simulink model "sampleModel191"  (R2021b)
settings: Solver=VariableStepAuto  StartTime=0.0  StopTime=10.0  RelTol=1e-3
libraries: simulink x2
settings Model: Creator=user  LastModifiedBy=user

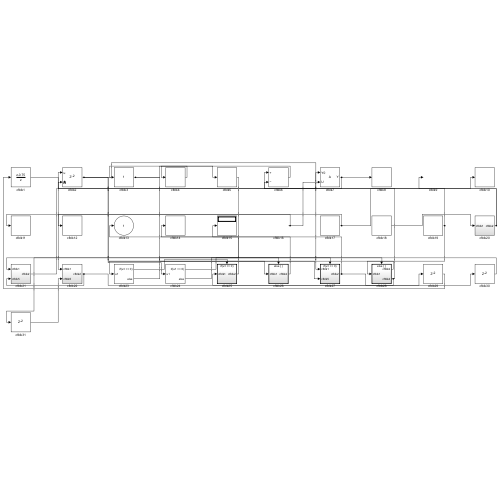
[thumbnail: Simulink's stored preview of the top-level diagram]
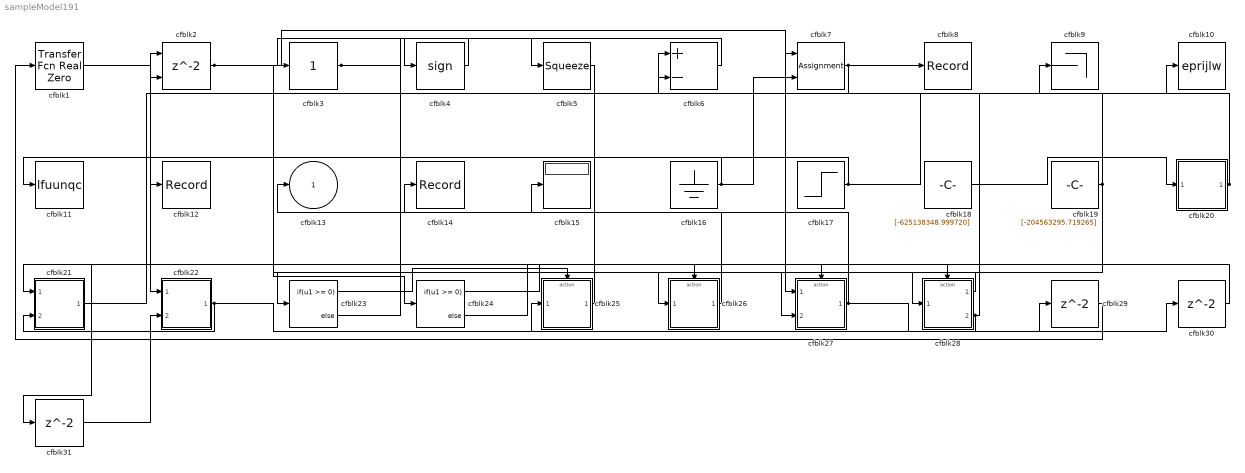
== system sampleModel191 ==
  cfblk1 : simulink/Discrete/Transfer Fcn Real Zero  ZeroZ=0.75  ICPrevInput=0.0  DoSatur=off
      settings: SourceProductBaseCode=SL
  cfblk10 : ToWorkspace  VariableName=eprijlw  SaveFormat=Timeseries  SampleTime=-1
  cfblk11 : ToWorkspace  VariableName=lfuunqc  SaveFormat=Timeseries  SampleTime=-1
  cfblk12 : Record  FileSettingsInternal="{\"entries\":[{\"content\":{\"excelSettings\":{\"content\":{},\"type\":\"Streamout.ExcelSettings\"}},\"type\":\"Streamout.FileSettingStorage\",\"uuid\":\"be9789c7-0946-41dc-ba80-fdfecf057616\"}],\"packageUris\":[\"http://schema.mathworks.com/mf0/streamout_blocks/R2020a\"],\"version\":\"1.0\"}"  SignalsInternal="{\"entries\":[{\"content\":{\"signals\":[{\"content\":{\"blockPath\":[\"sampleModel191/cfblk12\"],\"channel\":[],\"dimensions\":[1],\"domain\":\"sampleModel191/cfblk12\",\"lineColor\":\"#77ac30\",\"plots\":[1],\"port\":1,\"sid\":[\"\"],\"signalID\":7140,\"signalName\":\"cfblk17\"},\"type\":\"RecordBlkView.Signal\",\"uuid\":\"3feb5f82-e466-445f-8270-1e8679e3d33b\"}]},\"type\":\"RecordBlkView.InputSignals\",\"uuid\":\"5d828b83-df96-49b2-94c2-6ae34a61bf7d\"}],\"packageUris\":[\"http://schema.mathworks.com/mf0/streamout_blocks/R2020a\"],\"version\":\"1.0\"}"  VisualizationBindings="{\"sparklinesplugin\":{\"info\":[{\"bindingParametersList\":[],\"subplotID\":1}]}}"
  cfblk14 : Record  FileSettingsInternal="{\"entries\":[{\"content\":{\"excelSettings\":{\"content\":{},\"type\":\"Streamout.ExcelSettings\"}},\"type\":\"Streamout.FileSettingStorage\",\"uuid\":\"e2498147-d1e1-4463-9837-c808039952d8\"}],\"packageUris\":[\"http://schema.mathworks.com/mf0/streamout_blocks/R2020a\"],\"version\":\"1.0\"}"  SignalsInternal="{\"entries\":[{\"content\":{\"signals\":[{\"content\":{\"blockPath\":[\"sampleModel191/cfblk14\"],\"channel\":[],\"dimensions\":[1],\"domain\":\"sampleModel191/cfblk14\",\"lineColor\":\"#edb120\",\"plots\":[1],\"port\":1,\"sid\":[\"\"],\"signalID\":7132,\"signalName\":\"cfblk25\"},\"type\":\"RecordBlkView.Signal\",\"uuid\":\"96d69e8b-c9dd-4632-86a4-9ef49d9a27d5\"}]},\"type\":\"RecordBlkView.InputSignals\",\"uuid\":\"17047321-6578-4322-be57-9c84a47ba275\"}],\"packageUris\":[\"http://schema.mathworks.com/mf0/streamout_blocks/R2020a\"],\"version\":\"1.0\"}"  VisualizationBindings="{\"sparklinesplugin\":{\"info\":[{\"bindingParametersList\":[],\"subplotID\":1}]}}"
  cfblk15 : Display
  cfblk16 : Ground
  cfblk17 : Step  Time=[11.000000]  Before=[445527667.725951]  After=[-252859869.067699]  SampleTime=0
  cfblk18 : Constant  Value=[-625138348.999720]  SampleTime=1
  cfblk19 : Constant  Value=[-204563295.719265]  SampleTime=1
  cfblk2 : Delay  ShowEnablePort=on  SampleTime=1
      settings: InputPortMap=u0,e6
  cfblk20 : Subsystem
  cfblk21 : Subsystem
  cfblk22 : Subsystem
  cfblk23 : If  IfExpression=u1 >= 0  SampleTime=1
  cfblk24 : If  IfExpression=u1 >= 0  SampleTime=1
  cfblk25 : Subsystem  TreatAsAtomicUnit=on
  cfblk26 : Subsystem  TreatAsAtomicUnit=on
  cfblk27 : Subsystem  TreatAsAtomicUnit=on
  cfblk28 : Subsystem  TreatAsAtomicUnit=on
  cfblk29 : Delay  SampleTime=1
  cfblk3 : simulink/Math Operations/Slider Gain  gain=1  low=0  high=2
  cfblk30 : Delay  SampleTime=1
  cfblk31 : Delay  SampleTime=1
  cfblk4 : Signum
  cfblk5 : Squeeze
  cfblk6 : Sum  Inputs=+-
  cfblk7 : Assignment  DiagnosticForDimensions=Warning  IndexOptions=Index vector (dialog)  Indices=1  OutputSizes=1
  cfblk8 : Record  FileSettingsInternal="{\"entries\":[{\"content\":{\"excelSettings\":{\"content\":{},\"type\":\"Streamout.ExcelSettings\"}},\"type\":\"Streamout.FileSettingStorage\",\"uuid\":\"bd7b378f-c1a3-4038-8272-f5a9bb60a3b8\"}],\"packageUris\":[\"http://schema.mathworks.com/mf0/streamout_blocks/R2020a\"],\"version\":\"1.0\"}"  SignalsInternal="{\"entries\":[{\"content\":{\"signals\":[{\"content\":{\"blockPath\":[\"sampleModel191/cfblk8\"],\"channel\":[],\"dimensions\":[1],\"domain\":\"sampleModel191/cfblk8\",\"lineColor\":\"#7e2f8e\",\"plots\":[1],\"port\":1,\"sid\":[\"\"],\"signalID\":7136,\"signalName\":\"cfblk7\"},\"type\":\"RecordBlkView.Signal\",\"uuid\":\"3014864a-0562-4ad7-a535-a08722fbc90b\"}]},\"type\":\"RecordBlkView.InputSignals\",\"uuid\":\"e5762ca2-eda9-4507-8338-dc4311cc2cab\"}],\"packageUris\":[\"http://schema.mathworks.com/mf0/streamout_blocks/R2020a\"],\"version\":\"1.0\"}"  VisualizationBindings="{\"sparklinesplugin\":{\"info\":[{\"bindingParametersList\":[],\"subplotID\":1}]}}"
  cfblk9 : Terminator
  cfblk13 : Outport
  wires:
  cfblk16/1 -> cfblk11/1, cfblk7/2
  cfblk26/1(cfblk2) -> cfblk15/1
  cfblk19/1 -> cfblk28/1(cfblk1), cfblk9/1
  cfblk6/1 -> cfblk4/1
  cfblk27/1(cfblk2) -> cfblk13/1, cfblk30/1
  cfblk1/1 -> cfblk22/1(cfblk1)
  cfblk3/1 -> cfblk26/1(cfblk1), cfblk5/1
  cfblk18/1 -> cfblk20/1(cfblk1)
  cfblk2/1 -> cfblk27/1(cfblk1), cfblk27/2(cfblk5), cfblk24/1
  cfblk4/1 -> cfblk3/1
  cfblk20/1(cfblk2) -> cfblk6/1, cfblk2/1
  cfblk17/1 -> cfblk12/1, cfblk10/1
  cfblk28/1(cfblk2) -> cfblk23/1
  cfblk25/1(cfblk2) -> cfblk14/1
  cfblk28/2(cfblk4) -> cfblk25/1(cfblk1), cfblk6/2
  cfblk7/1 -> cfblk8/1, cfblk2/2
  cfblk21/1(cfblk2) -> cfblk7/1
  cfblk22/1(cfblk2) -> cfblk21/2(cfblk5), cfblk29/1
  cfblk23/1 -> cfblk25/Action
  cfblk23/2 -> cfblk26/Action
  cfblk24/1 -> cfblk27/Action
  cfblk24/2 -> cfblk28/Action
  cfblk29/1 -> cfblk1/1
  cfblk30/1 -> cfblk21/1(cfblk1)
  cfblk5/1 -> cfblk31/1
  cfblk31/1 -> cfblk22/2(cfblk5)

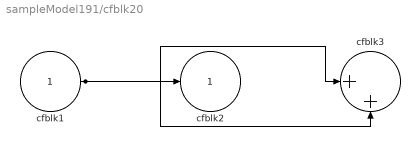
== system sampleModel191/cfblk20 ==
  cfblk1 : Inport
  cfblk3 : Sum  Inputs=|++
  cfblk2 : Outport
  wires:
  cfblk1/1 -> cfblk2/1, cfblk3/1, cfblk3/2

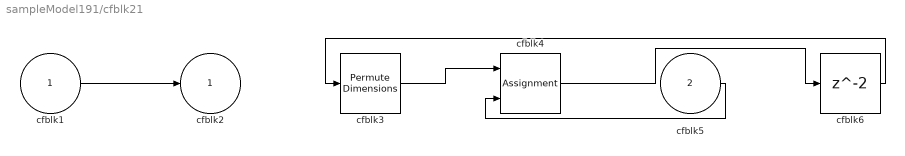
== system sampleModel191/cfblk21 ==
  cfblk1 : Inport
  cfblk5 : Inport  Port=2
  cfblk3 : PermuteDimensions
  cfblk4 : Assignment  DiagnosticForDimensions=Warning  IndexOptions=Index vector (dialog)  Indices=1  OutputSizes=1
  cfblk6 : Delay  SampleTime=1
  cfblk2 : Outport
  wires:
  cfblk1/1 -> cfblk2/1
  cfblk3/1 -> cfblk4/1
  cfblk5/1 -> cfblk4/2
  cfblk4/1 -> cfblk6/1
  cfblk6/1 -> cfblk3/1

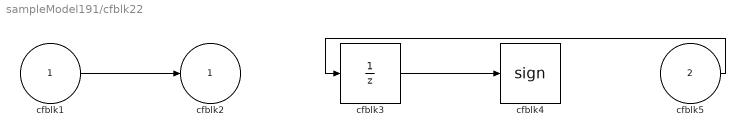
== system sampleModel191/cfblk22 ==
  cfblk1 : Inport
  cfblk5 : Inport  Port=2
  cfblk3 : UnitDelay  HasFrameUpgradeWarning=on
  cfblk4 : Signum
  cfblk2 : Outport
  wires:
  cfblk5/1 -> cfblk3/1
  cfblk1/1 -> cfblk2/1
  cfblk3/1 -> cfblk4/1

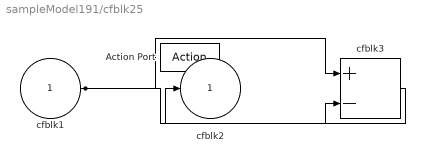
== system sampleModel191/cfblk25 ==
  cfblk1 : Inport
  Action Port : ActionPort  ActionPortLabel=if(u1 >= 0)
  cfblk3 : Sum  Inputs=+-
  cfblk2 : Outport
  wires:
  cfblk3/1 -> cfblk2/1
  cfblk1/1 -> cfblk3/1, cfblk3/2

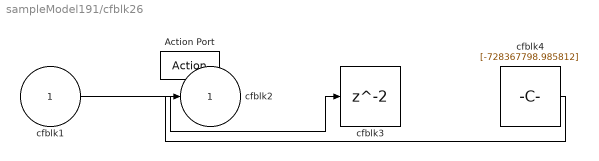
== system sampleModel191/cfblk26 ==
  cfblk1 : Inport
  Action Port : ActionPort  ActionPortLabel=else
  cfblk3 : Delay
  cfblk4 : Constant  Value=[-728367798.985812]  SampleTime=1
  cfblk2 : Outport
  wires:
  cfblk1/1 -> cfblk3/1
  cfblk4/1 -> cfblk2/1

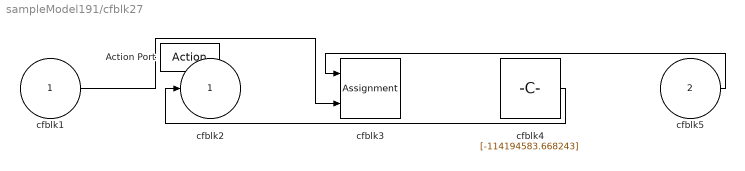
== system sampleModel191/cfblk27 ==
  cfblk1 : Inport
  cfblk5 : Inport  Port=2
  Action Port : ActionPort  ActionPortLabel=if(u1 >= 0)
  cfblk3 : Assignment  DiagnosticForDimensions=Warning  IndexOptions=Index vector (dialog)  Indices=1  OutputSizes=1
  cfblk4 : Constant  Value=[-114194583.668243]  SampleTime=1
  cfblk2 : Outport
  wires:
  cfblk5/1 -> cfblk3/1
  cfblk4/1 -> cfblk2/1
  cfblk1/1 -> cfblk3/2

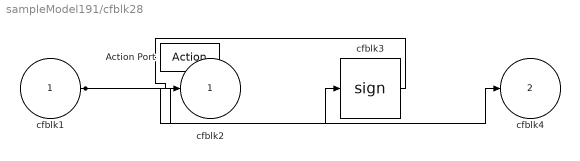
== system sampleModel191/cfblk28 ==
  cfblk1 : Inport
  Action Port : ActionPort  ActionPortLabel=else
  cfblk3 : Signum
  cfblk2 : Outport
  cfblk4 : Outport  Port=2
  wires:
  cfblk1/1 -> cfblk4/1, cfblk3/1
  cfblk3/1 -> cfblk2/1
